simulink model "SMA_spring_mass"  (R2018a)
settings: Solver=VariableStepAuto  StartTime=0.0  StopTime=30  RelTol=1e-3
undefined symbols (not defined in the file or in its folder): bias
settings Model: Creator=Matthias  LastModifiedBy=tim

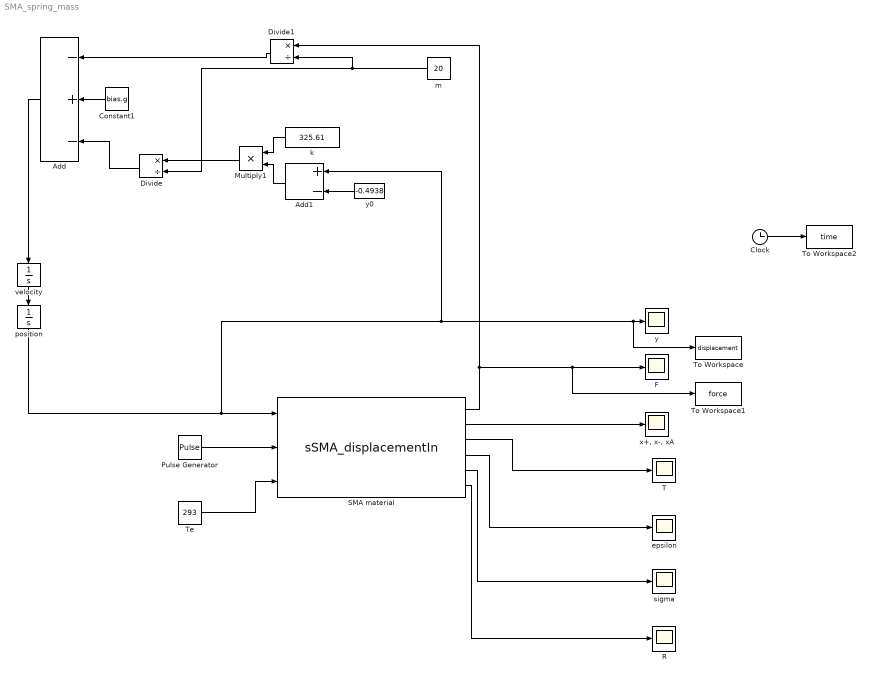
== system SMA_spring_mass ==
  Add : Sum  Inputs=-+-
  Add1 : Sum  Inputs=+-
  Clock : Clock
  Constant1 : Constant  Value=bias.g
  Divide : Product  Inputs=*/
  Divide1 : Product  Inputs=*/
  F : Scope
  Multiply1 : Product
  Pulse Generator : DiscretePulseGenerator  PulseType=Time based  Amplitude=0.4  Period=10  PulseWidth=50
  R : Scope
  SMA material : M-S-Function  FunctionName=sSMA_displacementIn  Parameters=params, initConds
      mask Display:
      | color('black');
      | patch(3*[-1 1 1 -1],1.1*[-1 -1 1 1],[1 1 1]);
      | patch([-1.6 -0.8],[-0.9 0.3],[0 0 0]);
      | patch([-0.8 1.2],[0.3 0.3],[0 0 0]);
      | patch([1.6 0.8],[0.9 -0.3],[0 0 0]);
      | patch([0.8 -1.2],[-0.3 -0.3],[0 0 0]);
      | disp('SMA');
      | 
      | color('blue');
      | port_label('input', 1, 'y [m]','texmode','on');
      | port_label('input', 2, 'J [W]','texmode','on');
      | port_label('input', 3, 'T_E [K]','texmode','on');
      | 
      | color('red');
      | port_label('output', 1, 'F [N]','texmode','on');
      | port_label('output', 2, 'x_+, x_-, x_A [-]','texmode','on');
      | port_label('output', 3, 'T [K]','texmode','on');
      | port_label('output', 4, '\epsilon [-]','texmode','on');
      | port_label('output', 5, '\sigma [Pa]','texmode','on');
      | port_label('output', 6, 'R [\Omega]','texmode','on');
  T : Scope
  Te : Constant  Value=293
  To Workspace : ToWorkspace  VariableName=displacement  SampleTime=-1
  To Workspace1 : ToWorkspace  VariableName=force  SampleTime=-1
  To Workspace2 : ToWorkspace  VariableName=time  SampleTime=-1
  epsilon : Scope
  k : Constant  Value=325.61
  m : Constant  Value=20
  position : Integrator  InitialCondition=bias.y0
  sigma : Scope
  velocity : Integrator  InitialCondition=bias.v0
  "x+, x-, xA" : Scope
  y : Scope
  y0 : Constant  Value=-0.4938
  wires:
  SMA material/2 -> "x+, x-, xA"/1
  Te/1 -> SMA material/3
  Pulse Generator/1 -> SMA material/2
  SMA material/6 -> R/1
  SMA material/3 -> T/1
  SMA material/5 -> sigma/1
  SMA material/4 -> epsilon/1
  SMA material/1 -> Divide1/1, To Workspace1/1, F/1
  Clock/1 -> To Workspace2/1
  velocity/1 -> position/1
  position/1 -> SMA material/1, Add1/1, To Workspace/1, y/1
  m/1 -> Divide/2, Divide1/2
  Add/1 -> velocity/1
  Divide1/1 -> Add/1
  y0/1 -> Add1/2
  Add1/1 -> Multiply1/2
  k/1 -> Multiply1/1
  Multiply1/1 -> Divide/1
  Divide/1 -> Add/3
  Constant1/1 -> Add/2
